simulink model "June30Simulink"  (R2015a)
settings: Solver=ode45  StartTime=0.0  StopTime=10.0  RelTol=1e-3
settings Model: Creator=admin  LastModifiedBy=admin

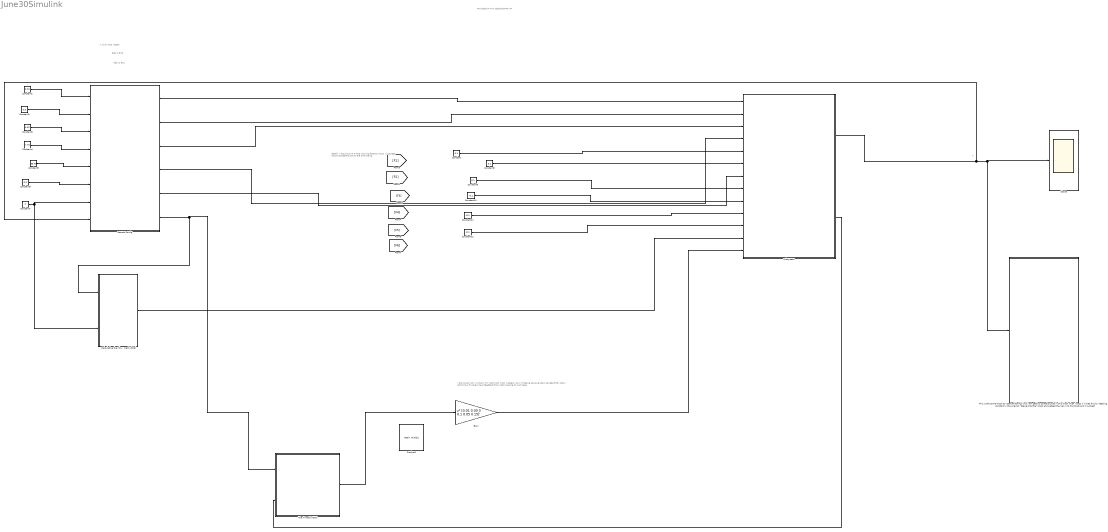
== system June30Simulink ==
  note: I should actually multiply H(X,Xdot) with Xdot.
      | Instead i am just taking some random constants for Xdot.
      | I dont know if just giving a feedback from Xdot is going to work here.
  note: M(X)Xddot + H(X,Xdot)Xdot =(J')*F
  note: X
  note: Ideally i should give
      | a time varying force as
      | input. I just kept it as a
      | constant(0.1N) for the time
      | being
  note: bdp is 3X1
  note: bRp is 3X3
  note: X is my 6X1 vector
  Calculating the Minv  matrix(6X6) : MATLAB Function  TreatAsAtomicUnit=on
  Constant : Constant  Value=0.1
  Constant1 : Constant  Value=0.10
  Constant10 : Constant  Value=-0.1
  Constant11 : Constant  Value=-0.1
  Constant12 : Constant  Value=-0.1
  Constant2 : Constant  Value=0.3
  Constant3 : Constant  Value=0.02
  Constant4 : Constant  Value=7.75
  Constant5 : Constant  Value=53.45
  Constant6 : Constant  Value=0.2
  Constant7 : Constant  Value=2
  Constant8 : Constant  Value=0.1
  Constant9 : Constant  Value=0.1
  Gain : Gain  Gain=[0.01 0.00 0 0.1 0.05 0.15]'  Multiplication=Matrix(u*K)
  Product1 : Product  Multiplication=Matrix(*)
  Scope : Scope
  Stewart Config : MATLAB Function  TreatAsAtomicUnit=on
  Subsystem : Subsystem
  The H matrix(6X6) : MATLAB Function  TreatAsAtomicUnit=on
  "This is the same block as \"Stewart Config\" but i am getting correct ouputs in this block when I pass X (I tried this by keeping X as constant in the original \"Stewart Config\" block and passed the new X to this block and it worked)" : MATLAB Function  TreatAsAtomicUnit=on
  wires:
  Constant1/1 -> Stewart Config/1(rp)
  Constant2/1 -> Stewart Config/2(rb)
  Constant3/1 -> Stewart Config/3(hp)
  Constant4/1 -> Stewart Config/4(gammap1)
  Constant5/1 -> Stewart Config/5(gammab1)
  Constant6/1 -> Stewart Config/6(vert)
  Constant7/1 -> Stewart Config/7(mplatform), Calculating the Minv  matrix(6X6)/2(mplatform)
  The H matrix(6X6)/1(H) -> Gain/1
  Stewart Config/6(bIp) -> The H matrix(6X6)/1(bIp), Calculating the Minv  matrix(6X6)/1(bIp)
  Subsystem/1(X(states)) -> Stewart Config/8(X), "This is the same block as \"Stewart Config\" but i am getting correct ouputs in this block when I pass X (I tried this by keeping X as constant in the original \"Stewart Config\" block and passed the new X to this block and it worked)"/1(X), Scope/1
  Stewart Config/1(bRp) -> Subsystem/1(bRp)
  Stewart Config/2(bdp) -> Subsystem/2(bdp)
  Stewart Config/3(bb) -> Subsystem/3(bb)
  Stewart Config/4(pp) -> Subsystem/4(pp)
  Constant/1 -> Subsystem/5(F1)
  Constant8/1 -> Subsystem/6(F2)
  Stewart Config/5(bA) -> Subsystem/7(bA)
  Constant9/1 -> Subsystem/8(F3)
  Constant10/1 -> Subsystem/9(F4)
  Constant11/1 -> Subsystem/10(F5)
  Constant12/1 -> Subsystem/11(F6)
  Calculating the Minv  matrix(6X6)/1(Minv) -> Subsystem/12(In12)
  Gain/1 -> Subsystem/13(In13)
  Subsystem/2(Xdot) -> The H matrix(6X6)/2(Xdot)

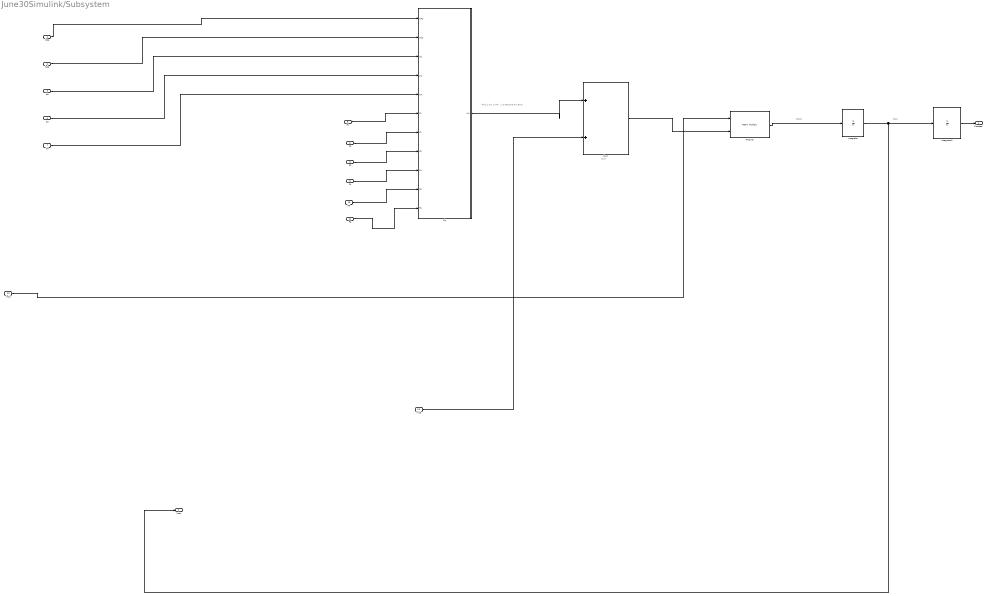
== system June30Simulink/Subsystem ==
  note: Xdot
  note: Xddot
  note: This is my (J')*F : ( J is 6X6 and F is 6X1)
  note: Sum
  bRp : Inport
  bdp : Inport  Port=2
  bb : Inport  Port=3
  pp : Inport  Port=4
  F1 : Inport  Port=5
  F2 : Inport  Port=6
  bA : Inport  Port=7
  F3 : Inport  Port=8
  F4 : Inport  Port=9
  F5 : Inport  Port=10
  F6 : Inport  Port=11
  In12 : Inport  Port=12
  In13 : Inport  Port=13
  Integrator : Integrator
  Integrator1 : Integrator
  Product : Product  Multiplication=Matrix(*)
  Sum : Sum  Inputs=|++
  Uin : MATLAB Function  TreatAsAtomicUnit=on
  X(states) : Outport
  Xdot : Outport  Port=2
  wires:
  F6/1 -> Uin/11(F6)
  F5/1 -> Uin/10(F5)
  bb/1 -> Uin/3(bb)
  bRp/1 -> Uin/1(bRp)
  Product/1 -> Integrator/1
  Uin/1(Uin) -> Sum/1
  F4/1 -> Uin/9(F4)
  In12/1 -> Product/1
  F3/1 -> Uin/8(F3)
  Sum/1 -> Product/2
  F1/1 -> Uin/6(F1)
  F2/1 -> Uin/7(F2)
  In13/1 -> Sum/2
  pp/1 -> Uin/4(pp)
  bdp/1 -> Uin/2(bdp)
  Integrator1/1 -> X(states)/1
  Integrator/1 -> Xdot/1, Integrator1/1
  bA/1 -> Uin/5(bA)

== matlab function June30Simulink/Stewart Config ==
  data: rp input; bRp output; rb input; hp input; gammap1 input; gammab1 input; vert input; mplatform input; bdp output; bb output; pp output; bA output; bIp output; X input
function [bRp,bdp,bb,pp,bA,bIp] = fcn(rp,rb,hp,gammap1,gammab1,vert,mplatform,X)
%#codegen
%The states that were chosen were X=[x,y,z,phi,theta,psi] and
%X2=[xdot,ydot,zdot,p,q,r ]
%Due to this a  trnasformation matrix must be added to transform the body
%rates to Euler rates.
gammap = [gammap1,120-gammap1, 120+gammap1, -120-gammap1,-120+gammap1,-gammap1];
gammab = [gammab1,120-gammab1, 120+gammab1, -120-gammab1,-120+gammab1,-gammab1];

 %alphap = [0 , 120, 120, -120 , -120 , 0] ;  
 %betab = [60,60,180,180,-60,-60];
 

 % pIp = mplatform *[((rp^2)/4) , 0, 0; 0, ((rp*2)/4), 0; 0, 0, (rp^2)/2] ;
    pp=zeros(3,6);
    pp(1,: ) = rp*cos(gammap*pi/180);
    pp(2,: ) = rp*sin(gammap*pi/180) ;
    pp(3,: ) = [hp/2,hp/2,hp/2,hp/2,hp/2,hp/2 ] ;        %hp is the thickness of the platform
    bb=zeros(3,6);
    bb(1,: ) = rb*cos(gammab*pi/180);
    bb(2,: ) = rb*sin(gammab*pi/180);
    bb(3,: ) = [0 , 0, 0, 0 , 0, 0] ;
    
     bdp = [X(1,1);X(2,1); X(3,1)+vert];                       %Position of platform frame wrt base
     %bdp=[0.01,0.02,0.03+vert]';             %This was kept constant for testing in simulink model
    
    bDp = [bdp,bdp,bdp,bdp,bdp,bdp] ;                           %This is same for all 6 actuators
   
      psi=X(4,1);
      the=X(5,1);
      phi=X(6,1);
      %psi=0.0872;
      %the=0;
      %phi=0;
    
   
    spsi = sin(psi);
    cpsi = cos(psi);
    sthe = sin(the);
    cthe = cos(the);
    sphi = sin(phi);
    cphi = cos(phi);
    

    
    pIp = mplatform *[((0.15^2)/4) , 0, 0; 0, ((0.15*2)/4), 0; 0, 0, (0.15^2)/2] ;
    bRp=zeros(3,3);
    bRp(1,1 ) = cphi * cthe ;
    bRp(1,2 ) = -sphi*cpsi + cphi * sthe * spsi ;
    bRp(1,3 ) = sphi * spsi + cphi * sthe * cpsi ;
    bRp(2,1 ) = sphi * cthe ;
    bRp(2,2 ) = cphi * cpsi + sphi * sthe * spsi ;
    bRp(2,3 ) = -cphi * spsi + sphi * sthe * cpsi ;
    bRp(3,1 ) = -sthe ;
    bRp(3,2 ) = cthe * spsi ;
    bRp(3,3 ) = cthe * cpsi ;
    
     bA = bRp*pp + bDp - bb ;                                    %Actuator vector
    
     bIp=bRp*pIp*bRp';                                           %Inertia tensor varying due to orientation of platform wrt base
end

== matlab function June30Simulink/Subsystem/Uin ==
  data: bRp input; bdp input; bb input; Uin output; pp input; bA input; F1 input; F2 input; F3 input; F4 input; F5 input; F6 input
function Uin = fcn(bRp,bdp,bb,pp,bA,F1,F2,F3,F4,F5,F6)
%#codegen
    g=9.81;
    G=[0,0,-g]';
    Fvec=zeros(3,6);
    %We are going to add g in vector form to the input force
   %Uin=zeros(6,1);
    %for j=1:6
     %  Fvec(:,j)=F(j,a)*bA(:,j);
    %end
    Fvec(:,1)=F1*bA(:,1);
    Fvec(:,2)=F2*bA(:,2);
    Fvec(:,3)=F3*bA(:,3);
    Fvec(:,4)=F4*bA(:,4);
    Fvec(:,5)=F5*bA(:,5);
    Fvec(:,6)=F6*bA(:,6);
      
    
   U=zeros(6,1);                                              %Combined effect of gravity and force on actuators
     %for j=1:6
      % U(j,1)= F(j,a)+dot(Fvec(:,j),G);
     %end
     
     
     U(1,1)=F1+dot(Fvec(:,1),G);
     U(2,1)=F2+dot(Fvec(:,2),G);
     U(3,1)=F3+dot(Fvec(:,3),G);
     U(4,1)=F4+dot(Fvec(:,4),G);
     U(5,1)=F5+dot(Fvec(:,5),G);
     U(6,1)=F6+dot(Fvec(:,6),G);
    
     Jt=zeros(6,6);
   
      for i=1:6
      Jt(:,i ) = [ ( bRp*pp(:,i) + bdp - bb(:,i) ); cross( bRp*pp(:,i),bdp-bb(:,i) ) ] / norm(bA(:,i)) ;
  
      end
    
     Uin=Jt*U;                                                %Input u in state space form
end

== matlab function June30Simulink/Calculating the Minv  matrix(6X6) ==
  data: bIp input; mplatform input; Minv output
function Minv = fcn(bIp,mplatform)
%#codegen
%Minv=zeros(6,6);
m=mplatform*(eye(3));

z=zeros(3,3);
M=zeros(6,6);
Minv=zeros(6,6);
M=[m,z;z,bIp];
Minv=inv(M);
end

== matlab function June30Simulink/The H matrix(6X6) ==
  data: bIp input; H output; Xdot input
function H = fcn(bIp,Xdot)
%#codegen
%H=zeros(6,6);
bWp = [Xdot(4,1) ; Xdot(5,1) ; Xdot(6,1)] ;
%bWp=[0.1;0.05;0.15];
bWpskew=zeros(3,3);
bWpskew=[ 0 , -1*bWp(3,1) , bWp(2,1) ; 
         bWp(3,1) , 0 , -1*bWp(1,1)  ;
         -1*bWp(2,1), bWp(1,1), 0 ];
     z=zeros(3,3);
     h=zeros(3,3);
     h= bWpskew*bIp;                             %WxI 
    H=[z,z;z,h];
end

== matlab function June30Simulink/This is the same block as "Stewart Config" but i am getting correct ouputs in this block when I pass X (I tried this by keeping X as constant in the original "Stewart Config" block and passed the new X to this block and it worked) ==
  data: bRp output; bdp output; bb output; pp output; bA output; bIp output; X input
function [bRp,bdp,bb,pp,bA,bIp] = fcn(X)
%#codegen
%The states that were chosen were X=[x,y,z,phi,theta,psi] and
%X2=[xdot,ydot,zdot,p,q,r ]
%Due to this a  trnasformation matrix must be added to transform the body
%rates to Euler rates.
rp=0.15;
rb=0.30;
hp=0.01;
gammap1=7.75;
gammab1=53.45;
vert=0.2;
mplatform=2;

gammap = [gammap1,120-gammap1, 120+gammap1, -120-gammap1,-120+gammap1,-gammap1];
gammab = [gammab1,120-gammab1, 120+gammab1, -120-gammab1,-120+gammab1,-gammab1];


 %alphap = [0 , 120, 120, -120 , -120 , 0] ;  
 %betab = [60,60,180,180,-60,-60];
 

 % pIp = mplatform *[((rp^2)/4) , 0, 0; 0, ((rp*2)/4), 0; 0, 0, (rp^2)/2] ;
    pp=zeros(3,6);
    pp(1,: ) = rp*cos(gammap*pi/180);
    pp(2,: ) = rp*sin(gammap*pi/180) ;
    pp(3,: ) = [hp/2,hp/2,hp/2,hp/2,hp/2,hp/2 ] ;        %hp is the thickness of the platform
    bb=zeros(3,6);
    bb(1,: ) = rb*cos(gammab*pi/180);
    bb(2,: ) = rb*sin(gammab*pi/180);
    bb(3,: ) = [0 , 0, 0, 0 , 0, 0] ;
    
     bdp = [X(1,1),X(2,1),X(3,1)+vert]' ;                       %Position of platform frame wrt base
     %bdp=[0.01,0.02,0.03+vert]';
    bDp = [bdp,bdp,bdp,bdp,bdp,bdp] ;                           %This is same for all 6 actuators
   
      psi=X(4,1);
      the=X(5,1);
      phi=X(6,1);
      %psi=0.0872;
      %the=0;
      %phi=0;
    
   
    spsi = sin(psi);
    cpsi = cos(psi);
    sthe = sin(the);
    cthe = cos(the);
    sphi = sin(phi);
    cphi = cos(phi);
    

    
    pIp = mplatform *[((0.15^2)/4) , 0, 0; 0, ((0.15*2)/4), 0; 0, 0, (0.15^2)/2] ;
    bRp=zeros(3,3);
    bRp(1,1 ) = cphi * cthe ;
    bRp(1,2 ) = -sphi*cpsi + cphi * sthe * spsi ;
    bRp(1,3 ) = sphi * spsi + cphi * sthe * cpsi ;
    bRp(2,1 ) = sphi * cthe ;
    bRp(2,2 ) = cphi * cpsi + sphi * sthe * spsi ;
    bRp(2,3 ) = -cphi * spsi + sphi * sthe * cpsi ;
    bRp(3,1 ) = -sthe ;
    bRp(3,2 ) = cthe * spsi ;
    bRp(3,3 ) = cthe * cpsi ;
    
     bA = bRp*pp + bDp - bb ;                                    %Actuator vector
    
     bIp=bRp*pIp*bRp';                                           %Inertia tensor varying due to orientation of platform wrt base
end
